simulink model "MAS_2021_loic"  (R2024a)
settings: Solver=FixedStepAuto  StartTime=0.0  StopTime=3  FixedStep=1e-6  RelTol=1e-6
values from neighbouring files (symbols this model uses):
  abc_alpha_beta = sqrt(2/3) * [1, -1/2, -1/2 ... (first row only)    [main.m]
  Flux_1 = 1/(Msr^2 - Ls * Lr )  * [Rs*Lr, 0, -Rs*Msr, 0 ... (first row only)    [main.m]
  Flux_2 = 1/(Msr^2 - Ls * Lr )  * [0, 0, 0, 0 ... (first row only)    [main.m]
  frot = 0.01    [main.m]
  In = 8.3    [main.m]
  Inv_abc_alpha_beta = inv(abc_alpha_beta)    [main.m]
  Inv_Phi_Courant = inv(Phi_Courant)    [main.m]
  J = 0.025    [main.m]
  K_reg_flux = (2*xi_reg_flux*wo_reg_flux*Lr/Rr-1)/Msr    (= 8.40898232203)    [main.m]
  K_reg_vitesse = (2*xi_reg_vitesse*wo_reg_vitesse*T_meca-1)*frot    [main.m]
  ki = 2*wo_reg_courant*sigma*Ls*xi_reg-Rsr    [main.m]
  Kpi = ws*20    (= 6283.18530718)    [main.m]
  Lr = 0.194    [main.m]
  Ls = 0.182    [main.m]
  Msr = 0.182    [main.m]
  onduleur = V_MLI/3*[2,-1,-1 ... (first row only)    [main.m]
  p = 2    [main.m]
  Rr = 1.15    [main.m]
  Rsr = Rs+Rr*(Msr/Lr)^2    (= 2.61213200128)    [main.m]
  sigma = 1-Msr^2/(Ls*Lr)    (= 0.0618556701031)    [main.m]
  T_charge = 0    [main.m]
  T_MLI = 1/F_MLI    (= 0.0001)    [main.m]
  T_reg_flux = Msr*K_reg_flux*Lr/(Rr*wo_reg_flux^2)    (= 0.00458982566688)    [main.m]
  T_reg_vitesse = K_reg_vitesse/(T_meca*frot*wo_reg_vitesse^2)    [main.m]
  Tfiltre = 1e-5    (= 1e-05)    [main.m]
  Ti = ki/(wo_reg_courant^2*Ls*sigma)    [main.m]
  Tin = sqrt(10)/Kpi    [main.m]
  Trau = T_meca*1e-3    (= 0.0025)    [main.m]
  V_MLI = 540    [main.m]
  Vn = 380    [main.m]
  ws = 2*pi*Fn    (= 314.159265359)    [main.m]
libraries: slpidlib x10, simulink_extras x6, hdlsllib x3, simulink x3
(part 2 of 2)

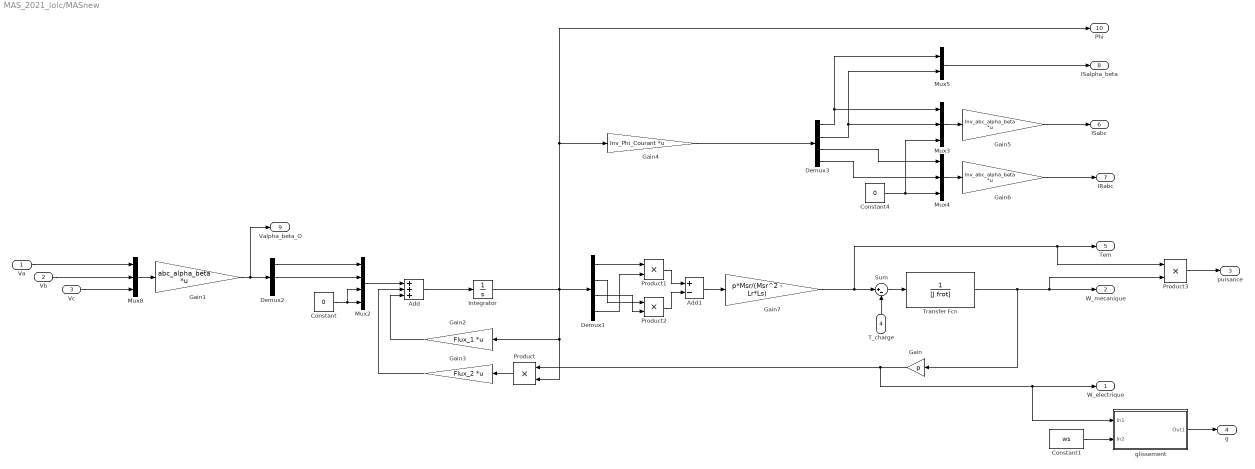
== system MAS_2021_loic/MASnew ==
  Va : Inport
  Vb : Inport  Port=2
  Vc : Inport  Port=3
  T_charge : Inport  Port=4
  Add : Sum  Inputs=+++
  Add1 : Sum  Inputs=+-
  Constant : Constant  Value=0
  Constant1 : Constant  Value=ws
  Constant4 : Constant  Value=0
  Demux1 : Demux
  Demux2 : Demux  Outputs=3
  Demux3 : Demux
  Gain : Gain  Gain=p
  Gain1 : Gain  Gain=abc_alpha_beta  Multiplication=Matrix(K*u)
  Gain2 : Gain  Gain=Flux_1  Multiplication=Matrix(K*u)
  Gain3 : Gain  Gain=Flux_2  Multiplication=Matrix(K*u)
  Gain4 : Gain  Gain=Inv_Phi_Courant  Multiplication=Matrix(K*u)
  Gain5 : Gain  Gain=Inv_abc_alpha_beta  Multiplication=Matrix(K*u)
  Gain6 : Gain  Gain=Inv_abc_alpha_beta  Multiplication=Matrix(K*u)
  Gain7 : Gain  Gain=p*Msr/(Msr^2 - Lr*Ls)
  Integrator : Integrator
  Mux2 : Mux
  Mux3 : Mux  Inputs=3
  Mux4 : Mux  Inputs=3
  Mux5 : Mux  Inputs=2
  Mux8 : Mux  Inputs=3
  Product{,1..3} (4 alike) : Product
  Sum : Sum  Inputs=|+-
  Transfer Fcn : TransferFcn  Denominator=[J frot]
  glissement : Subsystem
  W_electrique : Outport
  W_mecanique : Outport  Port=2
  puisance : Outport  Port=3
  g : Outport  Port=4
  Tem : Outport  Port=5
  ISabc : Outport  Port=6
  IRabc : Outport  Port=7
  ISalpha_beta : Outport  Port=8
  Valpha_beta_O : Outport  Port=9
  Phi : Outport  Port=10
  wires:
  Demux3/4 -> Mux4/2
  Demux3/2 -> Mux3/2, Mux5/2
  T_charge/1 -> Sum/2
  Demux3/1 -> Mux3/1, Mux5/1
  Va/1 -> Mux8/1
  Sum/1 -> Transfer Fcn/1
  Demux1/1 -> Product1/1
  Demux3/3 -> Mux4/1
  Gain7/1 -> Sum/1, Product3/1, Tem/1
  Transfer Fcn/1 -> Gain/1, Product3/2, W_mecanique/1
  Add/1 -> Integrator/1
  Vc/1 -> Mux8/3
  Vb/1 -> Mux8/2
  Product/1 -> Gain3/1
  Integrator/1 -> Gain2/1, Product/2, Demux1/1, Gain4/1, Phi/1
  Mux2/1 -> Add/1
  Mux3/1 -> Gain5/1
  Mux5/1 -> ISalpha_beta/1
  Gain1/1 -> Valpha_beta_O/1, Demux2/1
  Mux8/1 -> Gain1/1
  Demux2/1 -> Mux2/1
  Demux2/2 -> Mux2/2
  Constant/1 -> Mux2/4, Mux2/3
  Gain2/1 -> Add/3
  Gain4/1 -> Demux3/1
  Constant4/1 -> Mux4/3, Mux3/3
  Gain5/1 -> ISabc/1
  Mux4/1 -> Gain6/1
  Gain6/1 -> IRabc/1
  Product1/1 -> Add1/1
  Product2/1 -> Add1/2
  Add1/1 -> Gain7/1
  Gain/1 -> glissement/1(In1), W_electrique/1, Product/1
  Gain3/1 -> Add/2
  Demux1/4 -> Product1/2
  Demux1/2 -> Product2/1
  Demux1/3 -> Product2/2
  Product3/1 -> puisance/1
  glissement/1(Out1) -> g/1
  Constant1/1 -> glissement/2(In2)

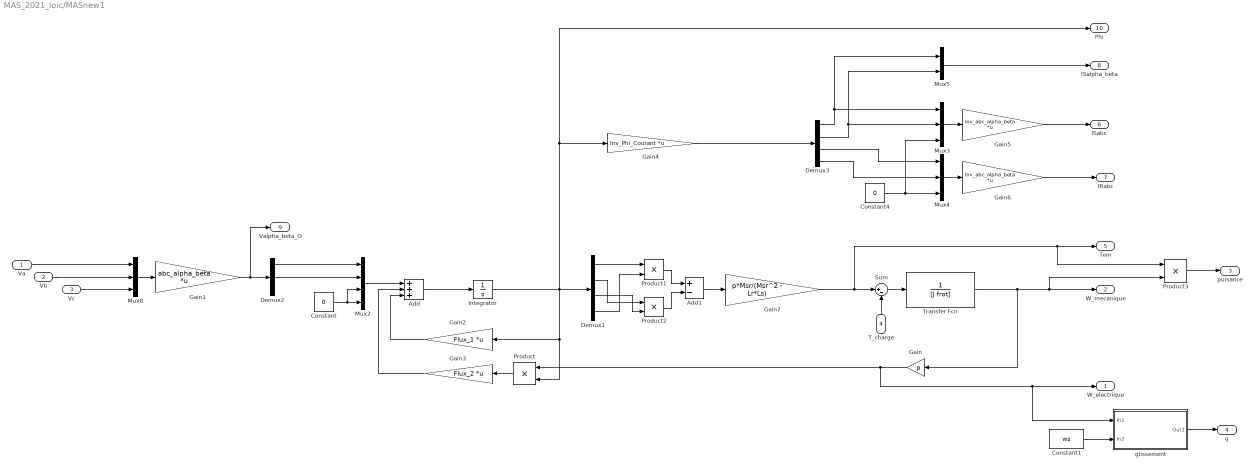
== system MAS_2021_loic/MASnew1 ==
  Va : Inport
  Vb : Inport  Port=2
  Vc : Inport  Port=3
  T_charge : Inport  Port=4
  Add : Sum  Inputs=+++
  Add1 : Sum  Inputs=+-
  Constant : Constant  Value=0
  Constant1 : Constant  Value=ws
  Constant4 : Constant  Value=0
  Demux1 : Demux
  Demux2 : Demux  Outputs=3
  Demux3 : Demux
  Gain : Gain  Gain=p
  Gain1 : Gain  Gain=abc_alpha_beta  Multiplication=Matrix(K*u)
  Gain2 : Gain  Gain=Flux_1  Multiplication=Matrix(K*u)
  Gain3 : Gain  Gain=Flux_2  Multiplication=Matrix(K*u)
  Gain4 : Gain  Gain=Inv_Phi_Courant  Multiplication=Matrix(K*u)
  Gain5 : Gain  Gain=Inv_abc_alpha_beta  Multiplication=Matrix(K*u)
  Gain6 : Gain  Gain=Inv_abc_alpha_beta  Multiplication=Matrix(K*u)
  Gain7 : Gain  Gain=p*Msr/(Msr^2 - Lr*Ls)
  Integrator : Integrator
  Mux2 : Mux
  Mux3 : Mux  Inputs=3
  Mux4 : Mux  Inputs=3
  Mux5 : Mux  Inputs=2
  Mux8 : Mux  Inputs=3
  Product{,1..3} (4 alike) : Product
  Sum : Sum  Inputs=|+-
  Transfer Fcn : TransferFcn  Denominator=[J frot]
  glissement : Subsystem
  W_electrique : Outport
  W_mecanique : Outport  Port=2
  puisance : Outport  Port=3
  g : Outport  Port=4
  Tem : Outport  Port=5
  ISabc : Outport  Port=6
  IRabc : Outport  Port=7
  ISalpha_beta : Outport  Port=8
  Valpha_beta_O : Outport  Port=9
  Phi : Outport  Port=10
  wires:
  Demux3/4 -> Mux4/2
  Demux3/2 -> Mux3/2, Mux5/2
  T_charge/1 -> Sum/2
  Demux3/1 -> Mux3/1, Mux5/1
  Va/1 -> Mux8/1
  Sum/1 -> Transfer Fcn/1
  Demux1/1 -> Product1/1
  Demux3/3 -> Mux4/1
  Gain7/1 -> Sum/1, Product3/1, Tem/1
  Transfer Fcn/1 -> Gain/1, Product3/2, W_mecanique/1
  Add/1 -> Integrator/1
  Vc/1 -> Mux8/3
  Vb/1 -> Mux8/2
  Product/1 -> Gain3/1
  Integrator/1 -> Gain2/1, Product/2, Demux1/1, Gain4/1, Phi/1
  Mux2/1 -> Add/1
  Mux3/1 -> Gain5/1
  Mux5/1 -> ISalpha_beta/1
  Gain1/1 -> Valpha_beta_O/1, Demux2/1
  Mux8/1 -> Gain1/1
  Demux2/1 -> Mux2/1
  Demux2/2 -> Mux2/2
  Constant/1 -> Mux2/4, Mux2/3
  Gain2/1 -> Add/3
  Gain4/1 -> Demux3/1
  Constant4/1 -> Mux4/3, Mux3/3
  Gain5/1 -> ISabc/1
  Mux4/1 -> Gain6/1
  Gain6/1 -> IRabc/1
  Product1/1 -> Add1/1
  Product2/1 -> Add1/2
  Add1/1 -> Gain7/1
  Gain/1 -> glissement/1(In1), W_electrique/1, Product/1
  Gain3/1 -> Add/2
  Demux1/4 -> Product1/2
  Demux1/2 -> Product2/1
  Demux1/3 -> Product2/2
  Product3/1 -> puisance/1
  glissement/1(Out1) -> g/1
  Constant1/1 -> glissement/2(In2)

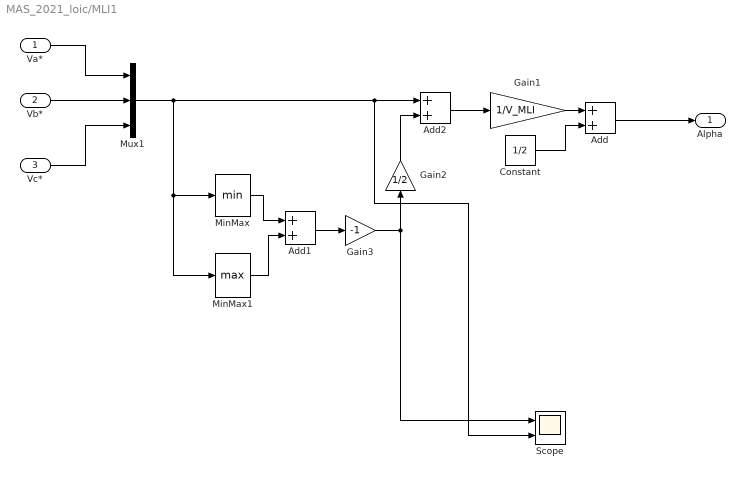
== system MAS_2021_loic/MLI1 ==
  Va* : Inport
  Vb* : Inport  Port=2
  Vc* : Inport  Port=3
  Add : Sum
  Add1 : Sum
  Add2 : Sum
  Constant : Constant  Value=1/2
  Gain1 : Gain  Gain=1/V_MLI
  Gain2 : Gain  Gain=1/2
  Gain3 : Gain  Gain=-1
  MinMax : MinMax
  MinMax1 : MinMax  Function=max
  Mux1 : Mux  Inputs=3
  Scope : Scope  NumInputPorts=2
  Alpha : Outport
  wires:
  Va*/1 -> Mux1/1
  Gain1/1 -> Add/1
  Vb*/1 -> Mux1/2
  Vc*/1 -> Mux1/3
  Add/1 -> Alpha/1
  Add2/1 -> Gain1/1
  Constant/1 -> Add/2
  Gain2/1 -> Add2/2
  Mux1/1 -> Add2/1, Scope/2, MinMax/1, MinMax1/1
  Add1/1 -> Gain3/1
  MinMax/1 -> Add1/1
  MinMax1/1 -> Add1/2
  Gain3/1 -> Scope/1, Gain2/1

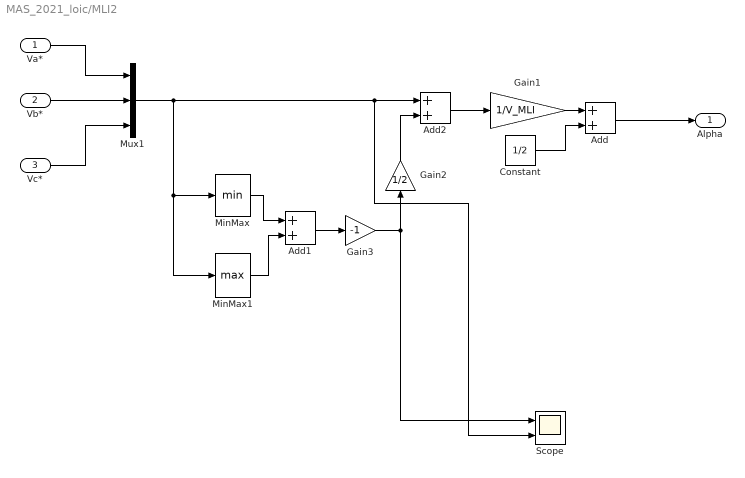
== system MAS_2021_loic/MLI2 ==
  Va* : Inport
  Vb* : Inport  Port=2
  Vc* : Inport  Port=3
  Add : Sum
  Add1 : Sum
  Add2 : Sum
  Constant : Constant  Value=1/2
  Gain1 : Gain  Gain=1/V_MLI
  Gain2 : Gain  Gain=1/2
  Gain3 : Gain  Gain=-1
  MinMax : MinMax
  MinMax1 : MinMax  Function=max
  Mux1 : Mux  Inputs=3
  Scope : Scope  NumInputPorts=2
  Alpha : Outport
  wires:
  Va*/1 -> Mux1/1
  Gain1/1 -> Add/1
  Vb*/1 -> Mux1/2
  Vc*/1 -> Mux1/3
  Add/1 -> Alpha/1
  Add2/1 -> Gain1/1
  Constant/1 -> Add/2
  Gain2/1 -> Add2/2
  Mux1/1 -> Add2/1, Scope/2, MinMax/1, MinMax1/1
  Add1/1 -> Gain3/1
  MinMax/1 -> Add1/1
  MinMax1/1 -> Add1/2
  Gain3/1 -> Scope/1, Gain2/1

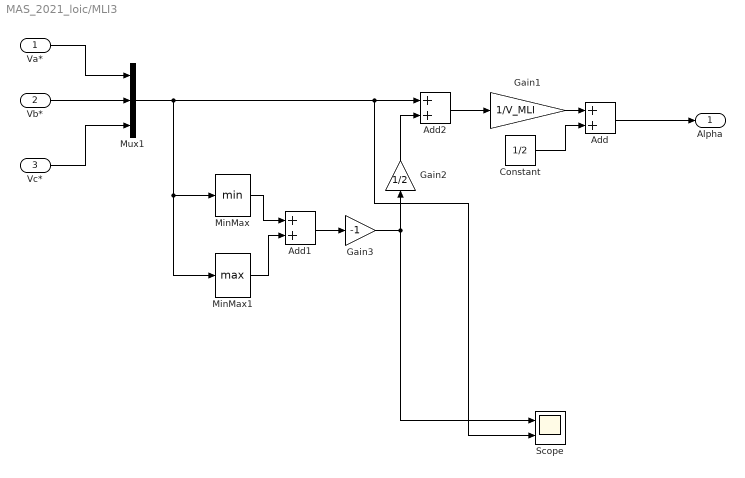
== system MAS_2021_loic/MLI3 ==
  Va* : Inport
  Vb* : Inport  Port=2
  Vc* : Inport  Port=3
  Add : Sum
  Add1 : Sum
  Add2 : Sum
  Constant : Constant  Value=1/2
  Gain1 : Gain  Gain=1/V_MLI
  Gain2 : Gain  Gain=1/2
  Gain3 : Gain  Gain=-1
  MinMax : MinMax
  MinMax1 : MinMax  Function=max
  Mux1 : Mux  Inputs=3
  Scope : Scope  NumInputPorts=2
  Alpha : Outport
  wires:
  Va*/1 -> Mux1/1
  Gain1/1 -> Add/1
  Vb*/1 -> Mux1/2
  Vc*/1 -> Mux1/3
  Add/1 -> Alpha/1
  Add2/1 -> Gain1/1
  Constant/1 -> Add/2
  Gain2/1 -> Add2/2
  Mux1/1 -> Add2/1, Scope/2, MinMax/1, MinMax1/1
  Add1/1 -> Gain3/1
  MinMax/1 -> Add1/1
  MinMax1/1 -> Add1/2
  Gain3/1 -> Scope/1, Gain2/1

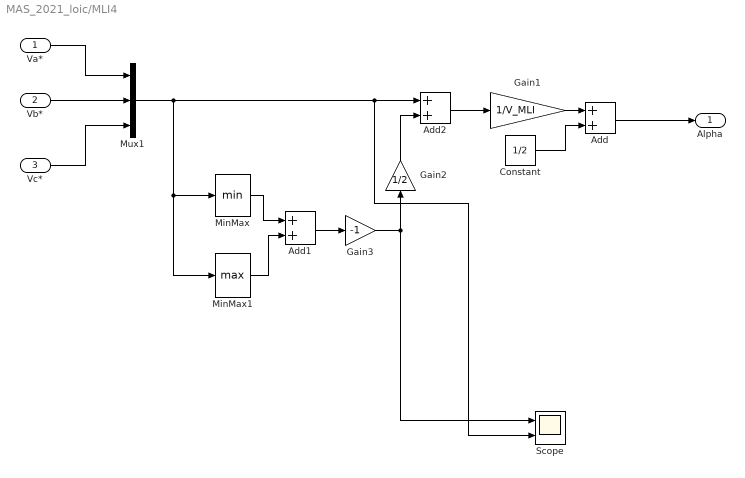
== system MAS_2021_loic/MLI4 ==
  Va* : Inport
  Vb* : Inport  Port=2
  Vc* : Inport  Port=3
  Add : Sum
  Add1 : Sum
  Add2 : Sum
  Constant : Constant  Value=1/2
  Gain1 : Gain  Gain=1/V_MLI
  Gain2 : Gain  Gain=1/2
  Gain3 : Gain  Gain=-1
  MinMax : MinMax
  MinMax1 : MinMax  Function=max
  Mux1 : Mux  Inputs=3
  Scope : Scope  NumInputPorts=2
  Alpha : Outport
  wires:
  Va*/1 -> Mux1/1
  Gain1/1 -> Add/1
  Vb*/1 -> Mux1/2
  Vc*/1 -> Mux1/3
  Add/1 -> Alpha/1
  Add2/1 -> Gain1/1
  Constant/1 -> Add/2
  Gain2/1 -> Add2/2
  Mux1/1 -> Add2/1, Scope/2, MinMax/1, MinMax1/1
  Add1/1 -> Gain3/1
  MinMax/1 -> Add1/1
  MinMax1/1 -> Add1/2
  Gain3/1 -> Scope/1, Gain2/1

== system MAS_2021_loic/Modulateur ==
  Alpha : Inport
  Add1 : Sum  Inputs=+-
  Compare To Zero : hdlsllib/Logic and Bit Operations/Compare To Zero  relop=>=  OutDataTypeStr=boolean
  Data Type Conversion : DataTypeConversion  SaturateOnIntegerOverflow=off  RndMeth=Floor
  Demux : Demux  Outputs=3
  Demux1 : Demux  Outputs=3
  Mux : Mux  Inputs=3
  Repeating Sequence : simulink/Sources/Repeating Sequence  rep_seq_t=[0 0.5*T_MLI T_MLI]  rep_seq_y=[1 0 1]
  Saturation : Saturate  UpperLimit=1  LowerLimit=0
  Scope : Scope
  commande : Outport
  wires:
  Alpha/1 -> Saturation/1
  Repeating Sequence/1 -> Mux/3, Add1/2
  Add1/1 -> Compare To Zero/1
  Saturation/1 -> Demux/1, Add1/1
  Compare To Zero/1 -> Data Type Conversion/1
  Data Type Conversion/1 -> Demux1/1, commande/1
  Mux/1 -> Scope/1
  Demux1/1 -> Mux/1
  Demux/1 -> Mux/2

== system MAS_2021_loic/Modulateur1 ==
  Alpha : Inport
  Add1 : Sum  Inputs=+-
  Compare To Zero : hdlsllib/Logic and Bit Operations/Compare To Zero  relop=>=  OutDataTypeStr=boolean
  Data Type Conversion : DataTypeConversion  SaturateOnIntegerOverflow=off  RndMeth=Floor
  Demux : Demux  Outputs=3
  Demux1 : Demux  Outputs=3
  Mux : Mux  Inputs=3
  Repeating Sequence : simulink/Sources/Repeating Sequence  rep_seq_t=[0 0.5*T_MLI T_MLI]  rep_seq_y=[1 0 1]
  Saturation : Saturate  UpperLimit=1  LowerLimit=0
  Scope : Scope
  commande : Outport
  wires:
  Alpha/1 -> Saturation/1
  Repeating Sequence/1 -> Mux/3, Add1/2
  Add1/1 -> Compare To Zero/1
  Saturation/1 -> Demux/1, Add1/1
  Compare To Zero/1 -> Data Type Conversion/1
  Data Type Conversion/1 -> Demux1/1, commande/1
  Mux/1 -> Scope/1
  Demux1/1 -> Mux/1
  Demux/1 -> Mux/2

== system MAS_2021_loic/Modulateur2 ==
  Alpha : Inport
  Add1 : Sum  Inputs=+-
  Compare To Zero : hdlsllib/Logic and Bit Operations/Compare To Zero  relop=>=  OutDataTypeStr=boolean
  Data Type Conversion : DataTypeConversion  SaturateOnIntegerOverflow=off  RndMeth=Floor
  Demux : Demux  Outputs=3
  Demux1 : Demux  Outputs=3
  Mux : Mux  Inputs=3
  Repeating Sequence : simulink/Sources/Repeating Sequence  rep_seq_t=[0 0.5*T_MLI T_MLI]  rep_seq_y=[1 0 1]
  Saturation : Saturate  UpperLimit=1  LowerLimit=0
  Scope : Scope
  commande : Outport
  wires:
  Alpha/1 -> Saturation/1
  Repeating Sequence/1 -> Mux/3, Add1/2
  Add1/1 -> Compare To Zero/1
  Saturation/1 -> Demux/1, Add1/1
  Compare To Zero/1 -> Data Type Conversion/1
  Data Type Conversion/1 -> Demux1/1, commande/1
  Mux/1 -> Scope/1
  Demux1/1 -> Mux/1
  Demux/1 -> Mux/2

== system MAS_2021_loic/Onduleur ==
  commande : Inport
  Demux : Demux  Outputs=3
  Gain : Gain  Gain=onduleur  Multiplication=Matrix(K*u)
  Va : Outport
  Vb : Outport  Port=2
  Vc : Outport  Port=3
  wires:
  Gain/1 -> Demux/1
  commande/1 -> Gain/1
  Demux/3 -> Vc/1
  Demux/1 -> Va/1
  Demux/2 -> Vb/1

== system MAS_2021_loic/Onduleur1 ==
  commande : Inport
  Demux : Demux  Outputs=3
  Gain : Gain  Gain=onduleur  Multiplication=Matrix(K*u)
  Va : Outport
  Vb : Outport  Port=2
  Vc : Outport  Port=3
  wires:
  Gain/1 -> Demux/1
  commande/1 -> Gain/1
  Demux/3 -> Vc/1
  Demux/1 -> Va/1
  Demux/2 -> Vb/1

== system MAS_2021_loic/Onduleur2 ==
  commande : Inport
  Demux : Demux  Outputs=3
  Gain : Gain  Gain=onduleur  Multiplication=Matrix(K*u)
  Va : Outport
  Vb : Outport  Port=2
  Vc : Outport  Port=3
  wires:
  Gain/1 -> Demux/1
  commande/1 -> Gain/1
  Demux/3 -> Vc/1
  Demux/1 -> Va/1
  Demux/2 -> Vb/1

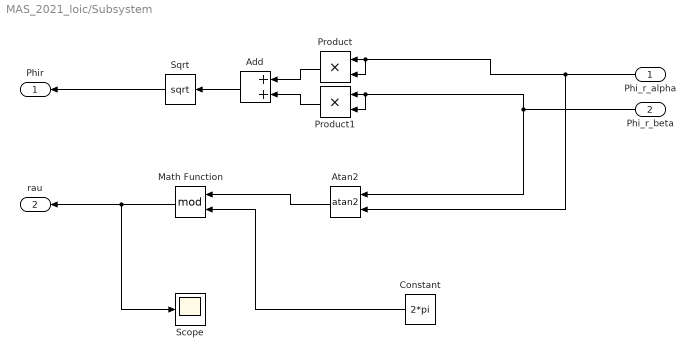
== system MAS_2021_loic/Subsystem ==
  Phi_r_alpha : Inport
  Phi_r_beta : Inport  Port=2
  Add : Sum
  Atan2 : Trigonometry  Operator=atan2
  Constant : Constant  Value=2*pi
  Math Function : Math  Operator=mod
  Product : Product
  Product1 : Product
  Scope : Scope
  Sqrt : Sqrt
  Phir : Outport
  rau : Outport  Port=2
  wires:
  Sqrt/1 -> Phir/1
  Product1/1 -> Add/2
  Add/1 -> Sqrt/1
  Phi_r_beta/1 -> Atan2/1, Product1/2, Product1/1
  Product/1 -> Add/1
  Phi_r_alpha/1 -> Atan2/2, Product/2, Product/1
  Atan2/1 -> Math Function/1
  Constant/1 -> Math Function/2
  Math Function/1 -> Scope/1, rau/1

== system MAS_2021_loic/Subsystem1 ==
  rau : Inport
  Constant : Constant  Value=2*pi
  Integrator : Integrator
  Mod : Math  Operator=mod
  Sum6 : Sum  Inputs=|+-
  Transfer Fcn1 : TransferFcn  Denominator=[Trau 1]
  Wrau : Outport
  wires:
  Constant/1 -> Mod/2
  Integrator/1 -> Mod/1
  Mod/1 -> Sum6/2
  Transfer Fcn1/1 -> Wrau/1, Integrator/1
  rau/1 -> Sum6/1
  Sum6/1 -> Transfer Fcn1/1

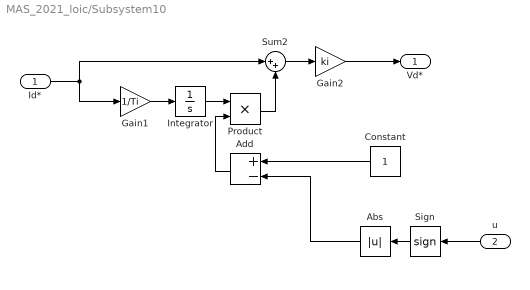
== system MAS_2021_loic/Subsystem10 ==
  Id* : Inport
  u : Inport  Port=2
  Abs : Abs  SaturateOnIntegerOverflow=off
  Add : Sum  Inputs=+-
  Constant : Constant
  Gain1 : Gain  Gain=1/Ti
  Gain2 : Gain  Gain=ki
  Integrator : Integrator
  Product : Product
  Sign : Signum
  Sum2 : Sum  Inputs=|++
  Vd* : Outport
  wires:
  Gain1/1 -> Integrator/1
  Integrator/1 -> Product/1
  Add/1 -> Product/2
  Sum2/1 -> Gain2/1
  Id*/1 -> Gain1/1, Sum2/1
  Product/1 -> Sum2/2
  Gain2/1 -> Vd*/1
  Sign/1 -> Abs/1
  Abs/1 -> Add/2
  Constant/1 -> Add/1
  u/1 -> Sign/1

== system MAS_2021_loic/Subsystem11 ==
  Iq* : Inport
  u : Inport  Port=2
  Abs : Abs  SaturateOnIntegerOverflow=off
  Add : Sum  Inputs=+-
  Constant : Constant
  Gain1 : Gain  Gain=1/Ti
  Gain2 : Gain  Gain=ki
  Integrator : Integrator
  Product : Product
  Sign : Signum
  Sum2 : Sum  Inputs=|++
  Vq* : Outport
  wires:
  Gain1/1 -> Integrator/1
  Integrator/1 -> Product/1
  Sum2/1 -> Gain2/1
  Iq*/1 -> Gain1/1, Sum2/1
  Product/1 -> Sum2/2
  Gain2/1 -> Vq*/1
  Constant/1 -> Add/1
  Add/1 -> Product/2
  u/1 -> Sign/1
  Sign/1 -> Abs/1
  Abs/1 -> Add/2

== system MAS_2021_loic/Subsystem12 ==
  Id* : Inport
  u : Inport  Port=2
  Abs : Abs  SaturateOnIntegerOverflow=off
  Add : Sum  Inputs=+-
  Constant : Constant
  Gain1 : Gain  Gain=1/Ti
  Gain2 : Gain  Gain=ki
  Integrator : Integrator
  Product : Product
  Sign : Signum
  Sum2 : Sum  Inputs=|++
  Vd* : Outport
  wires:
  Gain1/1 -> Integrator/1
  Integrator/1 -> Product/1
  Add/1 -> Product/2
  Sum2/1 -> Gain2/1
  Id*/1 -> Gain1/1, Sum2/1
  Product/1 -> Sum2/2
  Gain2/1 -> Vd*/1
  Sign/1 -> Abs/1
  Abs/1 -> Add/2
  Constant/1 -> Add/1
  u/1 -> Sign/1

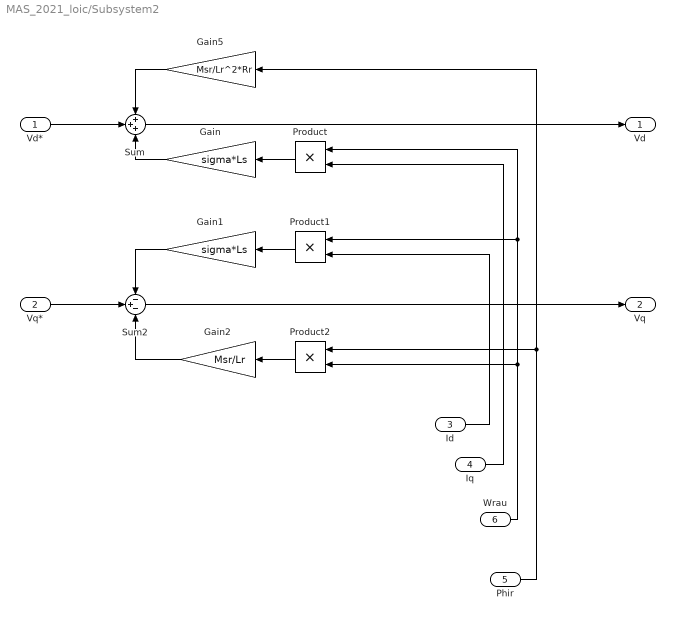
== system MAS_2021_loic/Subsystem2 ==
  Vd* : Inport
  Vq* : Inport  Port=2
  Id : Inport  Port=3
  Iq : Inport  Port=4
  Phir : Inport  Port=5
  Wrau : Inport  Port=6
  Gain : Gain  Gain=sigma*Ls
  Gain1 : Gain  Gain=sigma*Ls
  Gain2 : Gain  Gain=Msr/Lr
  Gain5 : Gain  Gain=Msr/Lr^2*Rr
  Product : Product
  Product1 : Product
  Product2 : Product
  Sum : Sum  Inputs=+++
  Sum2 : Sum  Inputs=-+-
  Vd : Outport
  Vq : Outport  Port=2
  wires:
  Vd*/1 -> Sum/2
  Iq/1 -> Product/2
  Id/1 -> Product1/2
  Gain/1 -> Sum/3
  Product/1 -> Gain/1
  Gain1/1 -> Sum2/1
  Product1/1 -> Gain1/1
  Vq*/1 -> Sum2/2
  Wrau/1 -> Product2/2, Product1/1, Product/1
  Phir/1 -> Product2/1, Gain5/1
  Gain5/1 -> Sum/1
  Sum2/1 -> Vq/1
  Product2/1 -> Gain2/1
  Sum/1 -> Vd/1
  Gain2/1 -> Sum2/3

== system MAS_2021_loic/Subsystem3 ==
  Id* : Inport
  u : Inport  Port=2
  Abs : Abs  SaturateOnIntegerOverflow=off
  Add : Sum  Inputs=+-
  Constant : Constant
  Gain1 : Gain  Gain=1/Ti
  Gain2 : Gain  Gain=ki
  Integrator : Integrator
  Product : Product
  Sign : Signum
  Sum2 : Sum  Inputs=|++
  Vd* : Outport
  wires:
  Gain1/1 -> Integrator/1
  Integrator/1 -> Product/1
  Add/1 -> Product/2
  Sum2/1 -> Gain2/1
  Id*/1 -> Gain1/1, Sum2/1
  Product/1 -> Sum2/2
  Gain2/1 -> Vd*/1
  Sign/1 -> Abs/1
  Abs/1 -> Add/2
  Constant/1 -> Add/1
  u/1 -> Sign/1

== system MAS_2021_loic/Subsystem4 ==
  Iq* : Inport
  u : Inport  Port=2
  Abs : Abs  SaturateOnIntegerOverflow=off
  Add : Sum  Inputs=+-
  Constant : Constant
  Gain1 : Gain  Gain=1/Ti
  Gain2 : Gain  Gain=ki
  Integrator : Integrator
  Product : Product
  Sign : Signum
  Sum2 : Sum  Inputs=|++
  Vq* : Outport
  wires:
  Gain1/1 -> Integrator/1
  Integrator/1 -> Product/1
  Sum2/1 -> Gain2/1
  Iq*/1 -> Gain1/1, Sum2/1
  Product/1 -> Sum2/2
  Gain2/1 -> Vq*/1
  Constant/1 -> Add/1
  Add/1 -> Product/2
  u/1 -> Sign/1
  Sign/1 -> Abs/1
  Abs/1 -> Add/2

== system MAS_2021_loic/Subsystem5 ==
  phir* : Inport
  u : Inport  Port=2
  Abs : Abs  SaturateOnIntegerOverflow=off
  Add : Sum  Inputs=+-
  Constant : Constant
  Gain1 : Gain  Gain=1/T_reg_flux
  Gain2 : Gain  Gain=K_reg_flux
  Integrator : Integrator
  Product : Product
  Sign : Signum
  Sum2 : Sum  Inputs=|++
  Id* : Outport
  wires:
  Gain1/1 -> Integrator/1
  Integrator/1 -> Product/1
  Add/1 -> Product/2
  Sum2/1 -> Gain2/1
  phir*/1 -> Sum2/1, Gain1/1
  Product/1 -> Sum2/2
  Gain2/1 -> Id*/1
  Sign/1 -> Abs/1
  Abs/1 -> Add/2
  Constant/1 -> Add/1
  u/1 -> Sign/1

== system MAS_2021_loic/Subsystem6 ==
  w* : Inport
  u : Inport  Port=2
  Abs : Abs  SaturateOnIntegerOverflow=off
  Add : Sum  Inputs=+-
  Constant : Constant
  Gain1 : Gain  Gain=1/T_reg_vitesse
  Gain2 : Gain  Gain=K_reg_vitesse
  Integrator : Integrator
  Product : Product
  Sign : Signum
  Sum2 : Sum  Inputs=|++
  Ce* : Outport
  wires:
  Gain1/1 -> Integrator/1
  Integrator/1 -> Product/1
  Sum2/1 -> Gain2/1
  w*/1 -> Gain1/1, Sum2/1
  Product/1 -> Sum2/2
  Gain2/1 -> Ce*/1
  Constant/1 -> Add/1
  Add/1 -> Product/2
  u/1 -> Sign/1
  Sign/1 -> Abs/1
  Abs/1 -> Add/2

== system MAS_2021_loic/Subsystem7 ==
  Phi_r_alpha : Inport
  Phi_r_beta : Inport  Port=2
  Add : Sum
  Atan2 : Trigonometry  Operator=atan2
  Constant : Constant  Value=2*pi
  Math Function : Math  Operator=mod
  Product : Product
  Product1 : Product
  Scope : Scope
  Sqrt : Sqrt
  Phir : Outport
  rau : Outport  Port=2
  wires:
  Sqrt/1 -> Phir/1
  Product1/1 -> Add/2
  Add/1 -> Sqrt/1
  Phi_r_beta/1 -> Atan2/1, Product1/2, Product1/1
  Product/1 -> Add/1
  Phi_r_alpha/1 -> Atan2/2, Product/2, Product/1
  Atan2/1 -> Math Function/1
  Constant/1 -> Math Function/2
  Math Function/1 -> Scope/1, rau/1

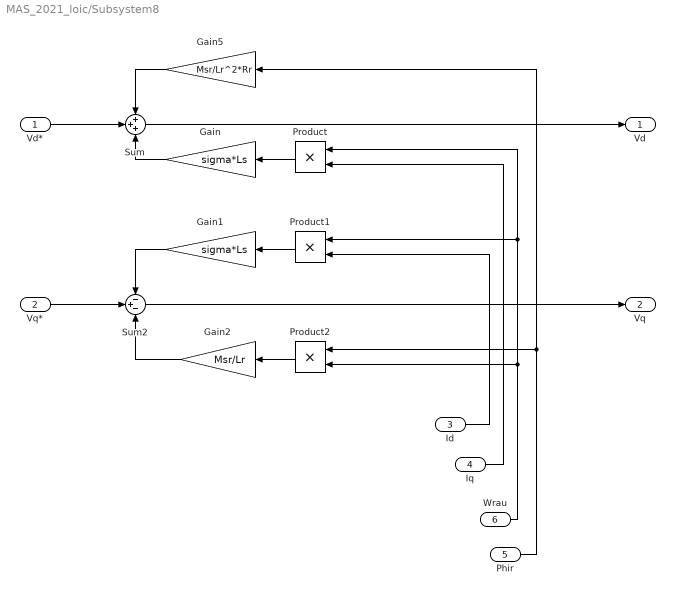
== system MAS_2021_loic/Subsystem8 ==
  Vd* : Inport
  Vq* : Inport  Port=2
  Id : Inport  Port=3
  Iq : Inport  Port=4
  Phir : Inport  Port=5
  Wrau : Inport  Port=6
  Gain : Gain  Gain=sigma*Ls
  Gain1 : Gain  Gain=sigma*Ls
  Gain2 : Gain  Gain=Msr/Lr
  Gain5 : Gain  Gain=Msr/Lr^2*Rr
  Product : Product
  Product1 : Product
  Product2 : Product
  Sum : Sum  Inputs=+++
  Sum2 : Sum  Inputs=-+-
  Vd : Outport
  Vq : Outport  Port=2
  wires:
  Vd*/1 -> Sum/2
  Iq/1 -> Product/2
  Id/1 -> Product1/2
  Gain/1 -> Sum/3
  Product/1 -> Gain/1
  Gain1/1 -> Sum2/1
  Product1/1 -> Gain1/1
  Vq*/1 -> Sum2/2
  Wrau/1 -> Product2/2, Product1/1, Product/1
  Phir/1 -> Product2/1, Gain5/1
  Gain5/1 -> Sum/1
  Sum2/1 -> Vq/1
  Product2/1 -> Gain2/1
  Sum/1 -> Vd/1
  Gain2/1 -> Sum2/3

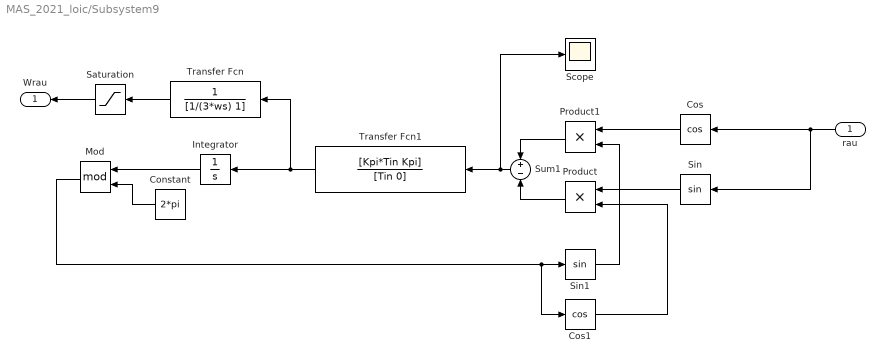
== system MAS_2021_loic/Subsystem9 ==
  rau : Inport
  Constant : Constant  Value=2*pi
  Cos : Trigonometry  Operator=cos
  Cos1 : Trigonometry  Operator=cos
  Integrator : Integrator
  Mod : Math  Operator=mod
  Product : Product
  Product1 : Product
  Saturation : Saturate  UpperLimit=1.2*ws  LowerLimit=-1.2*ws
  Scope : Scope
  Sin : Trigonometry
  Sin1 : Trigonometry
  Sum1 : Sum  Inputs=+|-
  Transfer Fcn : TransferFcn  Denominator=[1/(3*ws) 1]
  Transfer Fcn1 : TransferFcn  Numerator=[Kpi*Tin Kpi]  Denominator=[Tin 0]
  Wrau : Outport
  wires:
  Constant/1 -> Mod/2
  Integrator/1 -> Mod/1
  Mod/1 -> Cos1/1, Sin1/1
  Sum1/1 -> Scope/1, Transfer Fcn1/1
  rau/1 -> Sin/1, Cos/1
  Sin/1 -> Product/1
  Cos/1 -> Product1/1
  Sin1/1 -> Product1/2
  Cos1/1 -> Product/2
  Product1/1 -> Sum1/1
  Product/1 -> Sum1/2
  Transfer Fcn/1 -> Saturation/1
  Transfer Fcn1/1 -> Transfer Fcn/1, Integrator/1
  Saturation/1 -> Wrau/1

== system MAS_2021_loic/anti-windup ==
  x : Inport
  y : Inport  Port=2
  Cartesian to Polar : simulink_extras/Transformations/Cartesian to Polar
  Polar to Cartesian : simulink_extras/Transformations/Polar to Cartesian
  Saturation4 : Saturate  UpperLimit=V_MLI/sqrt(3)  LowerLimit=0
  Sum2 : Sum  Inputs=+|-
  Sum3 : Sum  Inputs=+|-
  x1 : Outport
  y1 : Outport  Port=2
  Out4 : Outport  Port=3
  Out1 : Outport  Port=4
  wires:
  Polar to Cartesian/2 -> y1/1, Sum3/2
  Polar to Cartesian/1 -> x1/1, Sum2/2
  x/1 -> Cartesian to Polar/1, Sum2/1
  Sum2/1 -> Out1/1
  y/1 -> Cartesian to Polar/2, Sum3/1
  Cartesian to Polar/1 -> Saturation4/1
  Saturation4/1 -> Polar to Cartesian/1
  Cartesian to Polar/2 -> Polar to Cartesian/2
  Sum3/1 -> Out4/1

== system MAS_2021_loic/anti-windup2 ==
  x : Inport
  y : Inport  Port=2
  Cartesian to Polar : simulink_extras/Transformations/Cartesian to Polar
  Polar to Cartesian : simulink_extras/Transformations/Polar to Cartesian
  Saturation4 : Saturate  UpperLimit=1.15*In  LowerLimit=0
  Sum2 : Sum  Inputs=+|-
  Sum3 : Sum  Inputs=+|-
  x1 : Outport
  y1 : Outport  Port=2
  u : Outport  Port=3
  Out1 : Outport  Port=4
  wires:
  Polar to Cartesian/2 -> y1/1, Sum3/2
  Polar to Cartesian/1 -> x1/1, Sum2/2
  x/1 -> Cartesian to Polar/1, Sum2/1
  Sum2/1 -> Out1/1
  y/1 -> Cartesian to Polar/2, Sum3/1
  Cartesian to Polar/1 -> Saturation4/1
  Saturation4/1 -> Polar to Cartesian/1
  Cartesian to Polar/2 -> Polar to Cartesian/2
  Sum3/1 -> u/1

== system MAS_2021_loic/MASnew/glissement ==
  In1 : Inport
  In2 : Inport  Port=2
  Add2 : Sum  Inputs=+-
  Divide : Product  Inputs=*/
  Out1 : Outport
  wires:
  In2/1 -> Divide/2, Add2/1
  Divide/1 -> Out1/1
  In1/1 -> Add2/2
  Add2/1 -> Divide/1

== system MAS_2021_loic/MASnew1/glissement ==
  In1 : Inport
  In2 : Inport  Port=2
  Add2 : Sum  Inputs=+-
  Divide : Product  Inputs=*/
  Out1 : Outport
  wires:
  In2/1 -> Divide/2, Add2/1
  Divide/1 -> Out1/1
  In1/1 -> Add2/2
  Add2/1 -> Divide/1

== matlab function MAS_2021_loic/Transformée de Park-1 ==
  data: Vd input; Va output; Vb output; Vc output; Vq input; Vh input; rau input
function [Va, Vb, Vc] = dq_abc(Vd,Vq,Vh,rau)


    % Vecteur de tensions d'entrée
    V = [Vd;Vq;Vh];
    
    % Matrice de transformation
    transformation_matrix = 2/3 * [cos(rau), cos(rau - 2*pi/3), cos(rau + 2*pi/3);
                                         -sin(rau), -sin(rau - 2*pi/3), -sin(rau + 2*pi/3);
                                          1/sqrt(2), 1/sqrt(2), 1/sqrt(2)];
    
    % Calcul des résultats
    result = inv(transformation_matrix) * V;
    
    % Attribution des résultats aux sorties
    Va = result(1);
    Vb= result(2);
    Vc = result(3);




end

== matlab function MAS_2021_loic/Transformée de Park1 ==
  data: Ia input; Id output; Iq output; Ih output; Ib input; Ic input; rau input
function [Id,Iq,Ih] = dq_abc(Ia, Ib, Ic,rau)


    % Vecteur de tensions d'entrée
    I = [Ia; Ib; Ic];
    
    % Matrice de transformation
    transformation_matrix = 2/3 * [cos(rau), cos(rau - 2*pi/3), cos(rau + 2*pi/3);
                                         -sin(rau), -sin(rau - 2*pi/3), -sin(rau + 2*pi/3);
                                          1/sqrt(2), 1/sqrt(2), 1/sqrt(2)];
    
    % Calcul des résultats
    result = transformation_matrix * I;
    
    % Attribution des résultats aux sorties
    Id = result(1);
    Iq= result(2);
    Ih = result(3);




end

== matlab function MAS_2021_loic/Transformée de Park-2 ==
  data: Vd input; Va output; Vb output; Vc output; Vq input; Vh input; rau input
function [Va, Vb, Vc] = dq_abc(Vd,Vq,Vh,rau)


    % Vecteur de tensions d'entrée
    V = [Vd;Vq;Vh];
    
    % Matrice de transformation
    transformation_matrix = sqrt(2/3) * [cos(rau), cos(rau - 2*pi/3), cos(rau + 2*pi/3);
                                         -sin(rau), -sin(rau - 2*pi/3), -sin(rau + 2*pi/3);
                                          1/sqrt(2), 1/sqrt(2), 1/sqrt(2)];
    
    % Calcul des résultats
    result = inv(transformation_matrix) * V;
    
    % Attribution des résultats aux sorties
    Va = result(1);
    Vb= result(2);
    Vc = result(3);




end

== matlab function MAS_2021_loic/Transformée de Park ==
  data: Ia input; Id output; Iq output; Ih output; Ib input; Ic input; rau input
function [Id,Iq,Ih] = dq_abc(Ia, Ib, Ic,rau)


    % Vecteur de tensions d'entrée
    I = [Ia; Ib; Ic];
    
    % Matrice de transformation
    transformation_matrix = sqrt(2/3) * [cos(rau), cos(rau - 2*pi/3), cos(rau + 2*pi/3);
                                         -sin(rau), -sin(rau - 2*pi/3), -sin(rau + 2*pi/3);
                                          1/sqrt(2), 1/sqrt(2), 1/sqrt(2)];
    
    % Calcul des résultats
    result = transformation_matrix * I;
    
    % Attribution des résultats aux sorties
    Id = result(1);
    Iq= result(2);
    Ih = result(3);




end
